simulink model "TEST_LIDAR"  (R2022b)
settings: Solver=FixedStepAuto  StartTime=0.0  StopTime=inf  FixedStep=1e-3  RelTol=1e-3  EnableMultiTasking=on
model workspace (MAT data in the model file):
  SL_ROS_VariableLengthArrays_MaxSizes : object (value not decoded)
values from neighbouring files (symbols this model uses):
  data = theClient.GetLastFrameOfData()    [FuncMotive.m]
undefined symbols (not defined in the file or in its folder): angular, carstamp, CIRCUIT, CLTF_DAMP, CLTF_FREQ, CLTF_GAIN, CONTROL, CONTROL_INI, DiscIntNeverNeededParam, INPUT, linear, MCP3201, MD25, MODEL, MODEL_INI, mpcstate, MPU60X0, MPU9250, MSG, NAV_MPC_CONTROL, OUTPUT, RCRX, SAMPLING_TIME, SYSID_INPUT, VL6180X
libraries: raspberrypiCommlib x160, simulink x89, raspberrypiNetworklib x22, ros2lib x14, dspsigattribs x14, embedlinuxBasiclib x12, ctrlSharedLib x2, mpclib x1, vrlib x1, sldrtlib x1
(part 16 of 19)

== matlab function TEST_LIDAR/CONTROL/LOCAL TARGETS/NAVIGATION TARGETS/PATH PLANNER ==
  data: CONTROL_IN input Bus: CONTROL_Bus; CONTROL output Bus: CONTROL_Bus
function CONTROL = MPC_TARGET_UPDATE(CONTROL_IN)

%--------------------------------------------------------------
% COPY CONTROL BUS
%--------------------------------------------------------------
CONTROL = CONTROL_IN;

%--------------------------------------------------------------
% DISABLING TARGET UPDATE
%--------------------------------------------------------------
% CONTROL_STATUS
% / 0. INITIALIZATION     / 1. ESTIMATION    / 2. ACTIVE CONTROL
if CONTROL.STATE.CONTROL_STATUS < 2  % INITIALIZATION    
    return
end

%--------------------------------------------------------------
% TIME MANAGEMENT
%--------------------------------------------------------------
% Sampling time 
ts = CONTROL.PARAM.SAMPLING_TIME;
% Trajectory update time 
tc = 10*ts;
persistent initialize TIMER
if isempty(initialize)
    TIMER = 0;
    initialize = 1;
end
TIMER = TIMER + ts;
if TIMER > tc-ts/2
    TIMER = 0;
    return
end

%--------------------------------------------------------------
% PARAMETERS
%--------------------------------------------------------------
% Maximun velocity magnitude 
VEL_MAG_MAX = CONTROL.PARAM.VEL_MAG_MAX;
% Prediction horizon (<= prediction horizon in mpcDesigner)
P = 20;
% Circular outline radius
% WP_R = CONTROL.PARAM.WP_R;

%**************************************************************************

% Number of waypoints
NUM_WAYPOINTS = CONTROL.TARGET.MISSION_NUM_WAYPOINTS;
% Waypoint list
WP_LIST = CONTROL.TARGET.MISSION_WAYPOINTS(1:NUM_WAYPOINTS,:);
% Next waypoint
NEXT_WP = CONTROL.TARGET.MISSION_COUNT;
% TARGETS
CONTROL.TARGET.NAV_REF = CONTROL.TARGET.NAV_REF_LC;
CONTROL.TARGET.FORWARD_VEL_REF = CONTROL.TARGET.NAV_REF(1);
% Tolerances
WP_R = CONTROL.TARGET.MISSION_WP_RADIUS;
YA_ERR = CONTROL.TARGET.MISSION_YA_ERROR;
% POSITION UPDATE
POS_XY = CONTROL.INPUT.EARTH_POS(1:2);
YAW_ANG = CONTROL.INPUT.YAW_ANG;
POS_INC = (WP_LIST(NEXT_WP,2) - POS_XY(1)) + (WP_LIST(NEXT_WP,3) - POS_XY(2))*1i;
POS_INC_MAG = abs(POS_INC);
if POS_INC_MAG<WP_R
    if WP_LIST(NEXT_WP,1)>TIMER_NAV
        CONTROL.TARGET.FORWARD_VEL_REF = 0;
        CONTROL.TARGET.YAW_ANG_REF = WP_LIST(NEXT_WP,4)*pi/180;
        TIMER_NAV = TIMER_NAV + SAMPLING_TIME;
        if abs(CONTROL.TARGET.YAW_ANG_REF-YAW_ANG)>YA_ERR
            TIMER_NAV = 0;
        end
    else
        TIMER_NAV = 0;
        NEXT_WP = NEXT_WP + uint8(1);
        CONTROL.TARGET.FORWARD_VEL_REF = CONTROL.TARGET.NAV_REF(1);
        CONTROL.TARGET.YAW_ANG_REF = CONTROL.TARGET.NAV_REF(2);
    end
else
    CONTROL.TARGET.FORWARD_VEL_REF = CONTROL.TARGET.NAV_REF(1);
    CONTROL.TARGET.YAW_ANG_REF = CONTROL.TARGET.NAV_REF(2);
end
if NEXT_WP>size(WP_LIST,1)
    NEXT_WP = uint8(size(WP_LIST,1));
end
% CONTROL BUS UPDATE
CONTROL.TARGET.MISSION_COUNT = NEXT_WP;
CONTROL.TARGET.POS_XY_REF = WP_LIST(NEXT_WP,2:3)';
CONTROL.STATE.NEXT_WP = NEXT_WP;

%**************************************************************************            
VEL_XY = VEL_MAG_TARGET.*exp(1j*VEL_ANG_TARGET);
CONTROL.TARGET.VEL_XY_REF(1) = real(VEL_XY(1));
CONTROL.TARGET.VEL_XY_REF(2) = imag(VEL_XY(1));
CONTROL.TARGET.NAV_REF = [VEL_MAG_TARGET(1) ; VEL_ANG_TARGET(1)];

return

== matlab function TEST_LIDAR/GAZEBO SIMULATION/SENSORS/WALL RANGE SENSOR/ANGLE AND DISTANCE COMPUTATION/YAW_ANGLE_DISTANCE_COMPUTATION ==
  data: FRONT_DISTANCE input; CONTROL output Bus: CONTROL_Bus; REAR_DISTANCE input; CONTROL_IN input
function CONTROL = WALL_ORIENTATION(FRONT_DISTANCE,REAR_DISTANCE,CONTROL_IN)

%% UPDATE BUS
CONTROL = CONTROL_IN;
%% PARAMETERS
RANGE_SENS_DIST = CONTROL.PARAM.RANGE_SENS_DIST;
%% MEASUREMENTS
CONTROL.INPUT.RANGE_WALL_ANG = atan2((REAR_DISTANCE-FRONT_DISTANCE)/1000,RANGE_SENS_DIST);
CONTROL.INPUT.RANGE_WALL_DIST = (FRONT_DISTANCE+REAR_DISTANCE)/2*cos(CONTROL.INPUT.RANGE_WALL_ANG)/1000;
CONTROL.INPUT.RANGE_FRONT_DIST = FRONT_DISTANCE/1000; % m
CONTROL.INPUT.RANGE_REAR_DIST = REAR_DISTANCE/1000; % m

return

== matlab function TEST_LIDAR/CONTROL/LOCAL TARGETS/NAVIGATION TARGETS/TRAJECTORY PLANNER (POLYNOMIAL IN Vx & Vy) ==
  data: CONTROL_IN input Bus: CONTROL_Bus; CONTROL output Bus: CONTROL_Bus
function CONTROL = MPC_TARGET_UPDATE(CONTROL_IN)

%--------------------------------------------------------------
% COPY CONTROL BUS
%--------------------------------------------------------------
CONTROL = CONTROL_IN;

%--------------------------------------------------------------
% DISABLING TARGET UPDATE
%--------------------------------------------------------------
% CONTROL_STATUS
% / 0. INITIALIZATION     / 1. ESTIMATION    / 2. ACTIVE CONTROL
if CONTROL.STATE.CONTROL_STATUS < 2  % INITIALIZATION    
    return
end

%--------------------------------------------------------------
% TIME MANAGEMENT
%--------------------------------------------------------------
% Sampling time 
ts = CONTROL.PARAM.SAMPLING_TIME;
% Trajectory update time 
tc = 10*ts;
persistent initialize TIMER
if isempty(initialize)
    TIMER = 0;
    initialize = 1;
end
TIMER = TIMER + ts;
if TIMER > tc-ts/2
    TIMER = 0;
    return
end

%--------------------------------------------------------------
% PARAMETERS
%--------------------------------------------------------------
% Maximun velocity magnitude 
VEL_MAG_MAX = CONTROL.PARAM.VEL_MAG_MAX;
% Prediction horizon (<= prediction horizon in mpcDesigner)
P = 20;
% Circular outline radius
% WP_R = CONTROL.PARAM.WP_R;

%--------------------------------------------------------------
% MEASUREMENTS AND STATE
%--------------------------------------------------------------
VEL_MAG = CONTROL.INPUT.FORWARD_VEL;
VEL_ANG = CONTROL.INPUT.YAW_ANG;
VEL_X = CONTROL.INPUT.EARTH_VEL(1);
VEL_Y = CONTROL.INPUT.EARTH_VEL(2);
POS_XY = CONTROL.INPUT.EARTH_POS(1:2);
WP_XY = CONTROL.TARGET.MISSION_WAYPOINTS(1:CONTROL.TARGET.MISSION_NUM_WAYPOINTS,2:3)';
NEXT_WP = CONTROL.TARGET.MISSION_COUNT;
M = CONTROL.PARAM.NAV_MPC.PRED_HRZ;
if NEXT_WP == size(WP_XY,2)
    CONTROL.TARGET.NAV_REF_LC(1) = 0;
    CONTROL.TARGET.NAV_REF(1) = 0;
    CONTROL.TARGET.NAV_REF_MPC(1:M,1) = zeros(M,1);
    CONTROL.TARGET.VEL_XY_REF(1) = 0;
    CONTROL.TARGET.VEL_XY_REF(2) = 0;
    CONTROL.TARGET.FORWARD_VEL_REF = 0;
end

%--------------------------------------------------------------
% TRAJECTORY PLANNING
%--------------------------------------------------------------
% x(t) = sum(ai*t^i) i=0...N
% y(t) = sum(bi*t^i) i=0...N
% dx(t)/dt = vx(t) = sum(i*ai*t^(i-1)) i=0...N
% dy(t)/dt = vy(t) = sum(i*bi*t^(i-1)) i=0...N
% Position and distance data
pos_x = [POS_XY(1) WP_XY(1,NEXT_WP:end)]';
pos_y = [POS_XY(2) WP_XY(2,NEXT_WP:end)]'; 
d = abs(diff(pos_x) + 1j*diff(pos_y));
% Delete duplicated points (distance = 0)
ind = find(d>0);
pos_x = [pos_x(ind) ; pos_x(end)];
pos_y = [pos_y(ind) ; pos_y(end)];
d = abs(diff(pos_x) + 1j*diff(pos_y));
% Polynomial parameters
Np = min([4 length(pos_x)+1]);
% Polynomial order
N = Np-1;
% Parameter initialization
a = zeros(Np,1);
b = zeros(Np,1);
a(1) = pos_x(1);
b(1) = pos_y(1);
a(2) = VEL_X;
b(2) = VEL_Y;
% Time vector for target
t_tgt = (1:P)'*tc;
VEL_MAG_TARGET = zeros(P,1);
VEL_ANG_TARGET = zeros(P,1);
% Time matrix for velocity target computation
matTp = zeros(P,N+1);
matTv = zeros(P,N);
for nn = 1:N+1
    matTp(:,nn) = t_tgt.^(nn-1);
end
for nn = 1:N
    matTv(:,nn) = nn*t_tgt.^(nn-1);
end
flag_vel_max = true;
k = 1;
while flag_vel_max
    % Reaching time for the next waypoints
    t = cumsum([0 ; k*sqrt(2)*d(1:N-1)/VEL_MAG_MAX]);    
    % Polynomial coefficient estimation 
    % matBx = matA*a(3:Np);  
    % matBy = matA*b(3:Np)
    matA = zeros(Np-2);
    for nn = 1:Np-2
        matA(:,nn) = t(2:end).^(nn+1);
    end
    matBx = pos_x(2:Np-1) - a(2)*t(2:end) - a(1);
    matBy = pos_y(2:Np-1) - b(2)*t(2:end) - b(1);
    inv_matA = inv(matA);
    a(3:end) = inv_matA*matBx;
    b(3:end) = inv_matA*matBy;
    % Position target calculation
    px_tgt = matTp*a;
    py_tgt = matTp*b; 
    % Magnitude and angle velocity targets calculation
    vx_tgt = matTv*a(2:end);
    vy_tgt = matTv*b(2:end); 
    v_tgt = vx_tgt + 1j*vy_tgt;
    VEL_MAG_TARGET = abs(v_tgt);
    VEL_ANG_TARGET = angle(v_tgt)*(VEL_MAG_TARGET(1)>=0.005) + ...
                    VEL_ANG*ones(size(VEL_ANG_TARGET))*(VEL_MAG_TARGET(1)<0.005);
    % Decreasing velocity factor
    k = k*max(VEL_MAG_TARGET)/VEL_MAG_MAX;
    % Maximun velocity verification
    if (max(VEL_MAG_TARGET)/VEL_MAG_MAX)<=1.01
        flag_vel_max = false;
    end
end

%--------------------------------------------------------------
% UNWRAPPING
%--------------------------------------------------------------
aux1 = VEL_ANG_TARGET(1);
aux2 = VEL_ANG;
INC_VEL_ANG_TARGET = zeros(21,1);
INC_VEL_ANG_TARGET(1) = aux1-aux2;
for nn=1:10
    INC_VEL_ANG_TARGET(2*nn:2*nn+1) = [aux1-aux2-2*nn*pi ; aux1-aux2+2*nn*pi];
end
[~,ind] = min(abs(INC_VEL_ANG_TARGET));
VEL_ANG_TARGET(1) = aux2 + INC_VEL_ANG_TARGET(ind);
for nn = 2:P
    INC_VEL_ANG_TARGET = [VEL_ANG_TARGET(nn)-VEL_ANG_TARGET(nn-1)
                          VEL_ANG_TARGET(nn)-VEL_ANG_TARGET(nn-1)-2*pi
                          VEL_ANG_TARGET(nn)-VEL_ANG_TARGET(nn-1)+2*pi];
    [~,ind] = min(abs(INC_VEL_ANG_TARGET));
    VEL_ANG_TARGET(nn) = VEL_ANG_TARGET(nn-1) + INC_VEL_ANG_TARGET(ind);
end

%--------------------------------------------------------------
% CONTROL BUS UPDATE
%--------------------------------------------------------------
CONTROL.TARGET.NAV_REF_LC(1) = VEL_MAG_TARGET(1);
CONTROL.TARGET.NAV_REF_LC(2) = VEL_ANG_TARGET(1);
if M<=P
    CONTROL.TARGET.NAV_REF_MPC(1:M,1) = VEL_MAG_TARGET(1:M);
    CONTROL.TARGET.NAV_REF_MPC(1:M,2) = VEL_ANG_TARGET(1:M);
else
    CONTROL.TARGET.NAV_REF_MPC(1:M,1) = [VEL_MAG_TARGET(1:P); VEL_MAG_TARGET(end)*ones(M-P,1)];
    CONTROL.TARGET.NAV_REF_MPC(1:M,2) = [VEL_ANG_TARGET(1:P); VEL_ANG_TARGET(end)*ones(M-P,1)];
end
VEL_XY = VEL_MAG_TARGET.*exp(1j*VEL_ANG_TARGET);
CONTROL.TARGET.VEL_XY_REF(1) = real(VEL_XY(1));
CONTROL.TARGET.VEL_XY_REF(2) = imag(VEL_XY(1));
CONTROL.TARGET.NAV_REF = [VEL_MAG_TARGET(1) ; VEL_ANG_TARGET(1)];

return

== matlab function TEST_LIDAR/GAZEBO SIMULATION/SENSORS/READ MOTOR ENCODER/READ_ENCODER ==
  data: CONTROL_IN input Bus: CONTROL_Bus; right_enc input; CONTROL output Bus: CONTROL_Bus; left_enc input
function CONTROL = READ_ENCODER(CONTROL_IN,right_enc,left_enc)

%--------------------------------------------------------------
% UPDATE BUS
%--------------------------------------------------------------
CONTROL = CONTROL_IN;

%--------------------------------------------------------------
% STATE
%--------------------------------------------------------------
persistent initialize left_enc_prv right_enc_prv inc_com_ang_prv ...
           inc_dif_ang_prv inc2_com_ang_prv inc2_dif_ang_prv dif_ang ...
           dif_ang_offs left_enc_offs right_enc_offs

if isempty(initialize)
    left_enc_prv = zeros(2,1);
    right_enc_prv = zeros(2,1);
    left_enc_offs = 0;
    right_enc_offs = 0;
    inc_com_ang_prv = zeros(5,1);
    inc_dif_ang_prv = zeros(5,1);
    inc2_com_ang_prv = zeros(5,1);
    inc2_dif_ang_prv = zeros(5,1);
    dif_ang = 0;
    dif_ang_offs = 0;        
    initialize = 1;
end

%--------------------------------------------------------------
% PARAMETERS
%--------------------------------------------------------------
% Wheel gear ratio
WHEEL_GEAR_RATIO = CONTROL.PARAM.WHEEL_GEAR_RATIO;
% Motor gear ratio
MOTOR_GEAR_RATIO = CONTROL.PARAM.MOTOR_GEAR_RATIO;
% Encoder resolution: number of pulses / revolution of main shaft
MOTOR_ENC_RES = CONTROL.PARAM.MOTOR_ENC_RES; 

%--------------------------------------------------------------
% ENCODER READOUT
%--------------------------------------------------------------
right_enc = double(right_enc);
left_enc = double(left_enc); 
inc_right_enc = right_enc - right_enc_prv(1);
inc_left_enc = left_enc - left_enc_prv(1);
inc2_right_enc = right_enc - 2*right_enc_prv(1) + right_enc_prv(2);
inc2_left_enc = left_enc - 2*left_enc_prv(1) + left_enc_prv(2);
inc_right_ang = 360/MOTOR_ENC_RES/MOTOR_GEAR_RATIO/WHEEL_GEAR_RATIO*inc_right_enc;
inc_left_ang = 360/MOTOR_ENC_RES/MOTOR_GEAR_RATIO/WHEEL_GEAR_RATIO*inc_left_enc;
inc2_right_ang = 360/MOTOR_ENC_RES/MOTOR_GEAR_RATIO/WHEEL_GEAR_RATIO*inc2_right_enc;
inc2_left_ang = 360/MOTOR_ENC_RES/MOTOR_GEAR_RATIO/WHEEL_GEAR_RATIO*inc2_left_enc;
inc_com_ang = (inc_left_ang + inc_right_ang)/2;
inc_dif_ang = (inc_left_ang - inc_right_ang)/2;
inc2_com_ang = (inc2_left_ang + inc2_right_ang)/2;
inc2_dif_ang = (inc2_left_ang - inc2_right_ang)/2;
% Define first-order incremental encoder threshold 
THR_INC_ENC_DEG = 10; 
% Define second-order incremental encoder threshold 
THR_INC2_ENC_DEG = 1; 
% Check incremental limits
if (abs(inc_right_ang)>THR_INC_ENC_DEG)   || ...
   (abs(inc_left_ang)>THR_INC_ENC_DEG)    || ...
   (abs(inc2_right_ang)>THR_INC2_ENC_DEG) || ...
   (abs(inc2_left_ang)>THR_INC2_ENC_DEG)
    inc2_com_ang = mean(inc2_com_ang_prv);
    inc2_dif_ang = mean(inc2_dif_ang_prv);
    inc_com_ang = mean(inc_com_ang_prv) + inc2_com_ang;
    inc_dif_ang = mean(inc_dif_ang_prv) + inc2_dif_ang;
end
% Update differential angles
dif_ang = dif_ang + inc_dif_ang;
% Update previous values
left_enc_prv(2) = left_enc_prv(1);
right_enc_prv(2) = right_enc_prv(1);
left_enc_prv(1) = left_enc;
right_enc_prv(1) = right_enc;
inc_com_ang_prv = [inc_com_ang ; inc_com_ang_prv(1:end-1)];
inc_dif_ang_prv = [inc_dif_ang ; inc_dif_ang_prv(1:end-1)];
inc2_com_ang_prv = [inc2_com_ang ; inc2_com_ang_prv(1:end-1)];
inc2_dif_ang_prv = [inc2_dif_ang ; inc2_dif_ang_prv(1:end-1)];

%--------------------------------------------------------------
% CALIBRATION 
%--------------------------------------------------------------
ALFA_CALIB = 0.99;
if CONTROL.STATE.CURRENT_STATUS_SYS == 1  % CALIBRATION ENABLED
    dif_ang_offs  = ALFA_CALIB*dif_ang_offs  + (1-ALFA_CALIB)*dif_ang;
    left_enc_offs = ALFA_CALIB*left_enc_offs  + (1-ALFA_CALIB)*left_enc;
    right_enc_offs = ALFA_CALIB*right_enc_offs  + (1-ALFA_CALIB)*right_enc;
elseif CONTROL.STATE.CURRENT_STATUS_SYS == 0
    return
else
end 

%--------------------------------------------------------------
% ENCODER ANGLES
%--------------------------------------------------------------
CONTROL.INPUT.ENC_INC2_COM_ANG = inc2_com_ang;
CONTROL.INPUT.ENC_INC2_DIF_ANG = inc2_dif_ang;
CONTROL.INPUT.ENC_INC_COM_ANG = inc_com_ang;
CONTROL.INPUT.ENC_INC_DIF_ANG = inc_dif_ang;
CONTROL.INPUT.ENC_DIF_ANG = dif_ang-dif_ang_offs;
CONTROL.INPUT.ENC_MOTOR_ANG = 2*pi/MOTOR_ENC_RES/MOTOR_GEAR_RATIO/WHEEL_GEAR_RATIO*[left_enc-left_enc_offs right_enc-right_enc_offs]';

return

== matlab function TEST_LIDAR/GAZEBO SIMULATION/COMMUNICATIONS/TCP//IP LIDAR/NAV RX ==
  data: CONTROL_IN input; PAYLOAD input; CONTROL output Bus: CONTROL_Bus; STATUS input
function CONTROL  = NAV_DECODER(CONTROL_IN,PAYLOAD,STATUS)
% Initialization
CONTROL = CONTROL_IN;
%%%%%%%%%%%%%%%%%%%%%%%%%%%%%%%%%%%%%%%%%%%%%%%%%%%%%%%%%%%%%%%%%%%%%%%%%%%
% MCS MESSAGES
%%%%%%%%%%%%%%%%%%%%%%%%%%%%%%%%%%%%%%%%%%%%%%%%%%%%%%%%%%%%%%%%%%%%%%%%%%%
% WRITE IN THE CONTROL BUS
if STATUS==1
    for nn = 1:20
        CONTROL.INPUT.LIDAR_2D(nn,1) = double(typecast(PAYLOAD(8*nn-4:-1:8*(nn-1)+1),'single'));
        CONTROL.INPUT.LIDAR_2D(nn,2) = double(typecast(PAYLOAD(8*nn:-1:8*nn-3),'single'));
    end
end
%%%%%%%%%%%%%%%%%%%%%%%%%%%%%%%%%%%%%%%%%%%%%%%%%%%%%%%%%%%%%%%%%%%%%%%%%%%


return

== matlab function TEST_LIDAR/GAZEBO SIMULATION/SENSORS/READ MOTOR ENCODER/MATLAB Function ==
  data: right_enc input; avg_encoder output; left_enc input
function avg_encoder  = READ_ENCODER(right_enc,left_enc)


%--------------------------------------------------------------
% STATE
%--------------------------------------------------------------
persistent initialize left_enc_prv right_enc_prv avg_inc every_ten

if isempty(initialize)
    left_enc_prv = 0;
    right_enc_prv = 0;
    every_ten = 1;
    avg_inc = 0;
    initialize = 1;
end

%--------------------------------------------------------------
% ENCODER READOUT
%--------------------------------------------------------------
if (every_ten < 10)
    every_ten = every_ten+ 1;
else
    every_ten = 1;
    right_enc = double(right_enc);
    left_enc = double(left_enc); 
    inc_right_enc = right_enc - right_enc_prv;
    inc_left_enc = left_enc - left_enc_prv;
    avg_inc = (inc_left_enc + inc_right_enc)/2;
    
    % Update previous values
    left_enc_prv = left_enc;
    right_enc_prv = right_enc;
end


%--------------------------------------------------------------
% ENCODER ANGLES
%--------------------------------------------------------------
avg_encoder = avg_inc*2*pi/360/0.01;

return

== matlab function TEST_LIDAR/GAZEBO SIMULATION/COMMUNICATIONS/TCP//IP MCS/MCS RX ==
  data: CONTROL_IN input; PAYLOAD input; CONTROL output Bus: CONTROL_Bus; STATUS input
function CONTROL = MCS_DECODER(CONTROL_IN,PAYLOAD,STATUS)
% Initialization
CONTROL = CONTROL_IN;
%%%%%%%%%%%%%%%%%%%%%%%%%%%%%%%%%%%%%%%%%%%%%%%%%%%%%%%%%%%%%%%%%%%%%%%%%%%
% MCS MESSAGES
%%%%%%%%%%%%%%%%%%%%%%%%%%%%%%%%%%%%%%%%%%%%%%%%%%%%%%%%%%%%%%%%%%%%%%%%%%%

% CRC    
CRC_VALUE=uint16(65535);
for nn=1:24
    TMP=bitxor(uint16(PAYLOAD(nn)),bitand(CRC_VALUE,uint16(255)));
    TMP4=bitand(bitshift(TMP,4),uint16(255));
    TMP=bitxor(TMP,TMP4);
    TMP8=bitshift(TMP,8);
    TMP3=bitshift(TMP,3);
    TMP_4=bitshift(TMP,-4);
    CRC_VALUE=bitxor(bitshift(CRC_VALUE,-8),bitxor(TMP8,bitxor(TMP3,TMP_4)));
    CRC_VALUE=bitand(CRC_VALUE,uint16(65535));
end
CRC1=uint8(bitand(CRC_VALUE,uint16(255)));
CRC2=uint8(bitand(bitshift(CRC_VALUE,-8),uint16(255)));
% CRC checking
if (CRC1 == PAYLOAD(MESSAGE_LEN-1))  && (CRC2 == PAYLOAD(MESSAGE_LEN))
    % WRITE IN THE CONTROL BUS
    CONTROL.INPUT.MCS_EARTH_POS(1) = double(typecast(PAYLOAD(1:4),'single'));
    CONTROL.INPUT.MCS_EARTH_POS(2) = double(typecast(PAYLOAD(5:8),'single'));
    CONTROL.INPUT.MCS_EARTH_POS(3) = double(typecast(PAYLOAD(9:12),'single'));
    CONTROL.INPUT.MCS_EULER_ANG(1) = double(typecast(PAYLOAD(13:16),'single'));
    CONTROL.INPUT.MCS_EULER_ANG(2) = double(typecast(PAYLOAD(17:20),'single'));
    CONTROL.INPUT.MCS_EULER_ANG(3) = double(typecast(PAYLOAD(21:24),'single'));

    % UNWRAPPING
    aux1 = CONTROL.INPUT.MCS_EULER_ANG(3);
    aux2 = CONTROL.TARGET.YAW_ANG_REF;
    INC_ANG = zeros(41,1);
    INC_ANG(1) = aux1-aux2;
    for ii = 1:20
        INC_ANG(2*ii)   = aux1-aux2-2*ii*pi;
        INC_ANG(2*ii+1) = aux1-aux2+2*ii*pi;
    end
    [~,ind] = min(abs(INC_ANG));
    NAV_YAW_ANG = aux2 + INC_ANG(ind);
    CONTROL.INPUT.MCS_EULER_ANG(3) = NAV_YAW_ANG;

    % POSITION CORRECTION
    % rv = rm + rc*exp(Shi*j)
    % xv = xm + xc*cos(Shi);
    % yv = ym + yc*sin(Shi);
    CONTROL.INPUT.MCS_EARTH_POS(1) = CONTROL.INPUT.MCS_EARTH_POS(1) - CONTROL.PARAM.NAV_CENTER_POS(1)*cos(CONTROL.INPUT.MCS_EULER_ANG(3));
    CONTROL.INPUT.MCS_EARTH_POS(2) = CONTROL.INPUT.MCS_EARTH_POS(2) - CONTROL.PARAM.NAV_CENTER_POS(2)*sin(CONTROL.INPUT.MCS_EULER_ANG(3));

    % INITIAL POSITION COMPENSATION
    if CONTROL.STATE.CURRENT_STATUS_SYS>1
        CONTROL.INPUT.MCS_EARTH_POS = CONTROL.INPUT.MCS_EARTH_POS - CONTROL.PARAM.MCS_EARTH_POS_OFFS;
        CONTROL.INPUT.MCS_EULER_ANG = CONTROL.INPUT.MCS_EULER_ANG - CONTROL.PARAM.MCS_EULER_ANG_OFFS;
    end
    
end


return

== matlab function TEST_LIDAR/GAZEBO SIMULATION/COMMUNICATIONS/TCP//IP NAV/NAV RX ==
  data: CONTROL_IN input; PAYLOAD input; CONTROL output Bus: CONTROL_Bus; STATUS input
function CONTROL  = NAV_DECODER(CONTROL_IN,PAYLOAD,STATUS)
% Initialization
CONTROL = CONTROL_IN;
%%%%%%%%%%%%%%%%%%%%%%%%%%%%%%%%%%%%%%%%%%%%%%%%%%%%%%%%%%%%%%%%%%%%%%%%%%%
% MCS MESSAGES
%%%%%%%%%%%%%%%%%%%%%%%%%%%%%%%%%%%%%%%%%%%%%%%%%%%%%%%%%%%%%%%%%%%%%%%%%%%
% WRITE IN THE CONTROL BUS
if STATUS==1
    CONTROL.INPUT.NAV_EARTH_POS(1) = double(typecast(PAYLOAD(4:-1:1),'single'));
    CONTROL.INPUT.NAV_EARTH_POS(2) = double(typecast(PAYLOAD(8:-1:5),'single'));
    CONTROL.INPUT.NAV_EARTH_POS(3) = double(typecast(PAYLOAD(12:-1:9),'single'));
    CONTROL.INPUT.NAV_EULER_ANG(1) = double(typecast(PAYLOAD(16:-1:13),'single'));
    CONTROL.INPUT.NAV_EULER_ANG(2) = double(typecast(PAYLOAD(20:-1:17),'single'));
    CONTROL.INPUT.NAV_EULER_ANG(3) = double(typecast(PAYLOAD(24:-1:21),'single'));
    if CONTROL.STATE.CURRENT_STATUS_SYS>1
        CONTROL.INPUT.NAV_EARTH_POS = CONTROL.INPUT.NAV_EARTH_POS - CONTROL.PARAM.NAV_EARTH_POS_OFFS;
        CONTROL.INPUT.NAV_EULER_ANG = CONTROL.INPUT.NAV_EULER_ANG - CONTROL.PARAM.NAV_EULER_ANG_OFFS;
    end
end
% UNWRAPPING
aux1 = CONTROL.INPUT.NAV_EULER_ANG(3);
aux2 = CONTROL.INPUT.YAW_ANG;
INC_ANG = zeros(41,1);
INC_ANG(1) = aux1-aux2;
for ii = 1:20
    INC_ANG(2*ii)   = aux1-aux2-2*ii*pi;
    INC_ANG(2*ii+1) = aux1-aux2+2*ii*pi;
end
[~,ind] = min(abs(INC_ANG));
NAV_YAW_ANG = aux2 + INC_ANG(ind);
CONTROL.INPUT.NAV_EULER_ANG(3) = NAV_YAW_ANG;
%%%%%%%%%%%%%%%%%%%%%%%%%%%%%%%%%%%%%%%%%%%%%%%%%%%%%%%%%%%%%%%%%%%%%%%%%%%


return

== matlab function TEST_LIDAR/GAZEBO SIMULATION/COMMUNICATIONS/TCP//IP SLAM/SLAM TX ==
  data: CONTROL input Bus: CONTROL_Bus; PAYLOAD output
function PAYLOAD  = SLAM_CODER(CONTROL)

%--------------------------------------------------------------------------
% INITIALIZATION
%--------------------------------------------------------------------------
persistent init TIMER x y shi
if isempty(init)
    TIMER = 0;
    x = 0;
    y = 0;
    shi = 0;
    init = 1;
end

%--------------------------------------------------------------------------
% TIMER UPDATE
%--------------------------------------------------------------------------
ts = CONTROL.PARAM.SAMPLING_TIME;
TIMER = TIMER + ts;

%--------------------------------------------------------------------------
% FORWARD VELOCITY AND YAW RATE UPDATE
%--------------------------------------------------------------------------
v = CONTROL.INPUT.FORWARD_VELOCITY;
w = CONTROL.INPUT.YAW_RATE;

%--------------------------------------------------------------------------
% INTEGRATION
%--------------------------------------------------------------------------
shi = shi + w*ts;
vx = v*cos(shi);
vy = v*sin(shi);
x = x + vx*ts;
y = y + vy*ts;

if TIMER >= 0.1-ts/2
    % Payload definition
    PAYLOAD = [typecast(single(x),'uint8')'
               typecast(single(y),'uint8')'
               typecast(single(shi),'uint8')'];
    TIMER = 0;
    x = 0;
    y = 0;
    shi = 0;
else
    PAYLOAD = zeros(12,1,'uint8');
end

return

== matlab function TEST_LIDAR/GAZEBO SIMULATION/COMMUNICATIONS/UART_MUX/BT MCS/MCS RX ==
  data: CONTROL_IN input; BUFFER_RX_LAST input; CONTROL output Bus: CONTROL_Bus
function CONTROL  = MCS_DECODER(CONTROL_IN,BUFFER_RX_LAST)
                 
persistent BUFFER_RX 
if isempty(BUFFER_RX)
    BUFFER_RX = zeros(50,3,'uint8');
end

% Initialization
CONTROL = CONTROL_IN;
MESSAGE_LEN = 24;
[BUFFER_ROW,BUFFER_COL] = size(BUFFER_RX);
% Update buffer
BUFFER_RX_VEC = [BUFFER_RX(:) ; BUFFER_RX_LAST];
BUFFER_LEN = length(BUFFER_RX_VEC);
% Identify sequences [0 254]
IDX_AUX = find(BUFFER_RX_VEC(1:end-1)==uint8(0) & BUFFER_RX_VEC(2:end)==uint8(254));
if isempty(IDX_AUX) 
    % There is not any message
    BUFFER_RX = zeros(size(BUFFER_RX),'uint8');
    return
elseif IDX_AUX(1)+MESSAGE_LEN+1>BUFFER_LEN 
    % There is 1 incomplete message 
    BUFFER_RX = [BUFFER_RX(:,2:end)  BUFFER_RX_LAST];
    return
else
    % There is 1 complete message at least    
    IDX_START = zeros(size(IDX_AUX));
    IDX_END = zeros(size(IDX_AUX));
    IDX_AUX = [IDX_AUX ; BUFFER_LEN];
    IDX_START(1) = IDX_AUX(1) + 2;
    IDX_END(1) = IDX_START(1) + MESSAGE_LEN - 1;    
    COUNT = 1;
    % The rest of sequences [0 254] are verified
    for nn = 2:length(IDX_AUX)-1
        if (IDX_END(COUNT) < IDX_AUX(nn)) && (IDX_AUX(nn)+2<BUFFER_LEN)
            if IDX_AUX(nn) + MESSAGE_LEN + 1 <= BUFFER_LEN
                COUNT = COUNT +1;
                IDX_START(COUNT) = IDX_AUX(nn) + 2;
                IDX_END(COUNT) = IDX_START(COUNT) + MESSAGE_LEN - 1;       
            end
        end
    end
end
IDX_START = IDX_START(1:COUNT);
IDX_END = IDX_END(1:COUNT);
% Message identification
NUM_MESSAGES = COUNT;
MESSAGE = cell(NUM_MESSAGES,1);
for COUNT = 1:NUM_MESSAGES
    % Message building
    MESSAGE{COUNT} = BUFFER_RX_VEC(IDX_START(COUNT):IDX_END(COUNT));
end
% Update BUFFER_RX
BUFFER_RX_VEC = [zeros(IDX_END(end)-BUFFER_ROW-1,1,'uint8') ; BUFFER_RX_VEC(IDX_END(end):end)];
for nn = 1:BUFFER_COL
    BUFFER_RX(:,nn) = BUFFER_RX_VEC((nn-1)*BUFFER_ROW+1:BUFFER_ROW*nn);
end

%%%%%%%%%%%%%%%%%%%%%%%%%%%%%%%%%%%%%%%%%%%%%%%%%%%%%%%%%%%%%%%%%%%%%%%%%%%
% MCS MESSAGES
%%%%%%%%%%%%%%%%%%%%%%%%%%%%%%%%%%%%%%%%%%%%%%%%%%%%%%%%%%%%%%%%%%%%%%%%%%%
PAYLOAD = uint8(MESSAGE{end});

% Escribir en el bus de control
CONTROL.INPUT.MCS_POS_XY(1) = typecast(PAYLOAD(1:8),'double');
CONTROL.INPUT.MCS_POS_XY(2) = typecast(PAYLOAD(9:16),'double');
MCS_YAW_ANG = typecast(PAYLOAD(17:24),'double');
% UNWRAPPING
aux1 = MCS_YAW_ANG;
aux2 = CONTROL.TARGET.YAW_ANG_REF;
INC_YAW_ANG = [aux1-aux2
               aux1-aux2-2*pi
               aux1-aux2+2*pi];
[~,ind] = min(abs(INC_YAW_ANG));
MCS_YAW_ANG = aux2 + INC_YAW_ANG(ind);

CONTROL.INPUT.MCS_YAW_ANG = MCS_YAW_ANG;
%%%%%%%%%%%%%%%%%%%%%%%%%%%%%%%%%%%%%%%%%%%%%%%%%%%%%%%%%%%%%%%%%%%%%%%%%%%


return

== matlab function TEST_LIDAR/GAZEBO SIMULATION/COMMUNICATIONS/UART_MUX/MATLAB Function ==
  settings: updateMethod=DISCRETE  sampleTime=SAMPLING_TIME
  data: A output; B output; INH output; RCRX output; BL output
function [A,B,INH,RCRX,BL] = UART_MULTIPLEXER()

% Counter initialization
persistent initialize ii

if isempty(initialize)
    count = 0;
    initialize = true;
end

INH = false;
% Mux channel selection
switch count
    case 0
        A = false;
        B = false;
        BL = true;
        RCRX = false;
    case 1
        A = true;
        B = false;
        BL = false;
        RCRX = true;
    otherwise
        INH = true;
        A = false;
        B = false;
        BL = false;
        RCRX = false;
end
count = count + 1;
if count > 1 
    count = 0;
end
